simulink model "kaskada"  (Simulink 7.9)
settings: Solver=ode45  StartTime=0.0  StopTime=50.0  RelTol=1e-3
settings Model: Creator=student  LastModifiedBy=student

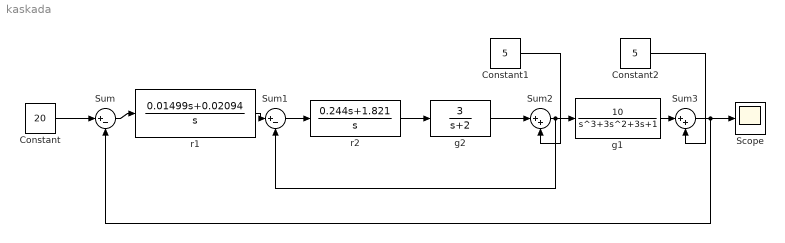
== system kaskada ==
  Constant : Constant  Value=20
  Constant1 : Constant  Value=5
  Constant2 : Constant  Value=5
  Scope : Scope
  Sum : Sum  Inputs=|+-
  Sum1 : Sum  Inputs=|+-
  Sum2 : Sum  Inputs=|++
  Sum3 : Sum  Inputs=|++
  g1 : TransferFcn  Numerator=[10]  Denominator=[1 3 3 1]
  g2 : TransferFcn  Numerator=[3]  Denominator=[1 2]
  r1 : TransferFcn  Numerator=[0.01499 0.02094]  Denominator=[1 0]
  r2 : TransferFcn  Numerator=[0.244 1.821]  Denominator=[1 0]
  wires:
  Constant/1 -> Sum/1
  Sum/1 -> r1/1
  r1/1 -> Sum1/1
  Sum1/1 -> r2/1
  r2/1 -> g2/1
  g2/1 -> Sum2/1
  Constant1/1 -> Sum2/2
  Sum2/1 -> g1/1, Sum1/2
  g1/1 -> Sum3/1
  Constant2/1 -> Sum3/2
  Sum3/1 -> Scope/1, Sum/2
